simulink model "Passband_modulation_techniques"  (R2018b)
settings: Solver=VariableStepAuto  StartTime=0.0  StopTime=0.1  RelTol=1e-3  EnableMultiTasking=on
libraries: commfilt2 x6, commutil2 x5, commrandsrc3 x4, simulink x4
settings Model: Creator=hp  LastModifiedBy=HP
settings OptimizationCC: LifeSpan=inf
settings DebuggingCC: SFUnexpectedBacktrackingDiag=warning  SFNoUnconditionalDefaultTransitionDiag=warning
settings SFSimCC: SimUseLocalCustomCode=off
settings RTWCC: RTWUseLocalCustomCode=off
settings CodeAppCC: StateflowObjectComments=on
settings GRTTargetCC: TargetLangStandard=C89/C90 (ANSI)
settings ConfigComp: CovMetricSettings=dw  CovHtmlReporting=on  CovSaveCumulativeToWorkspaceVar=on  CovSaveSingleToWorkspaceVar=on  CovExternalEMLEnable=off

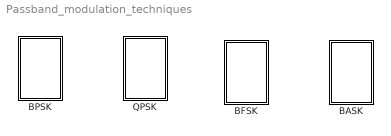
== system Passband_modulation_techniques ==
  BASK : Subsystem
  BFSK : Subsystem
  BPSK : Subsystem
  QPSK : Subsystem

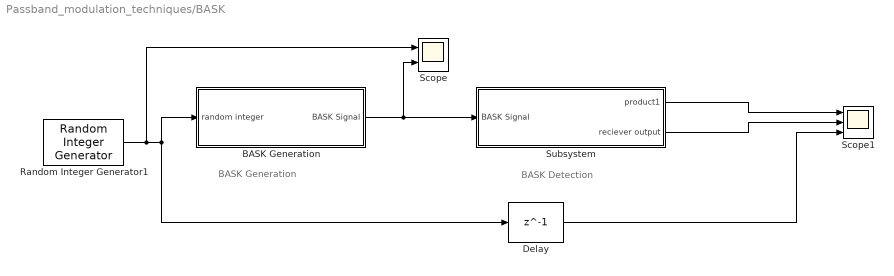
== system Passband_modulation_techniques/BASK ==
  note: BASK Detection
  note: BASK Generation
  BASK Generation : Subsystem
  Delay : Delay  DelayLength=1  InputProcessing=Columns as channels (frame based)
  Random Integer Generator1 : commrandsrc3/Random Integer Generator  SetSize=2  SeedSource=Auto  Seed=0  SampleTime=0.01  SamplesPerFrame=1  OutputDataType=double  SimulateUsing=Interpreted execution
  Scope : Scope  NumInputPorts=2
  Scope1 : Scope  NumInputPorts=3
  Subsystem : Subsystem
  wires:
  Subsystem/1(product1) -> Scope1/1
  Subsystem/2(reciever output) -> Scope1/2
  Delay/1 -> Scope1/3
  Random Integer Generator1/1 -> Scope/1, BASK Generation/1(random integer), Delay/1
  BASK Generation/1(BASK Signal) -> Scope/2, Subsystem/1(BASK Signal)

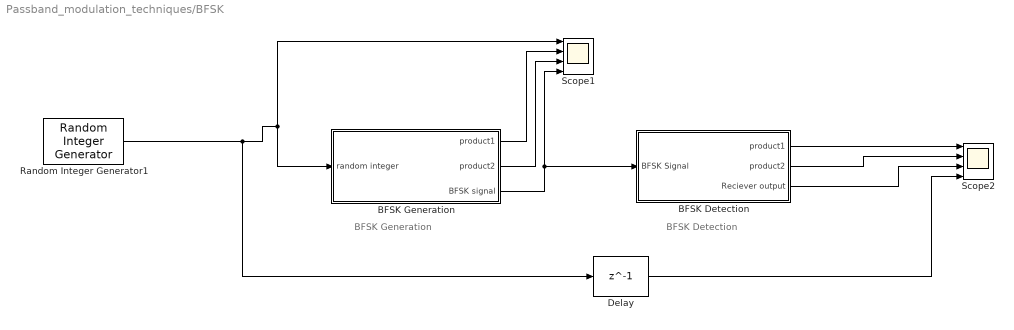
== system Passband_modulation_techniques/BFSK ==
  note: BFSK Detection
  note: BFSK Generation
  BFSK Detection : Subsystem
  BFSK Generation : Subsystem
  Delay : Delay  DelayLength=1  InputProcessing=Columns as channels (frame based)
  Random Integer Generator1 : commrandsrc3/Random Integer Generator  SetSize=2  SeedSource=Auto  Seed=0  SampleTime=0.01  SamplesPerFrame=1  OutputDataType=double  SimulateUsing=Interpreted execution
  Scope1 : Scope  NumInputPorts=4
  Scope2 : Scope  NumInputPorts=4
  wires:
  Random Integer Generator1/1 -> Delay/1, BFSK Generation/1(random integer), Scope1/1
  BFSK Generation/3(BFSK signal) -> Scope1/4, BFSK Detection/1(BFSK Signal)
  BFSK Generation/1(product1) -> Scope1/2
  BFSK Generation/2(product2) -> Scope1/3
  BFSK Detection/1(product1) -> Scope2/1
  BFSK Detection/2(product2) -> Scope2/2
  BFSK Detection/3(Reciever output) -> Scope2/3
  Delay/1 -> Scope2/4

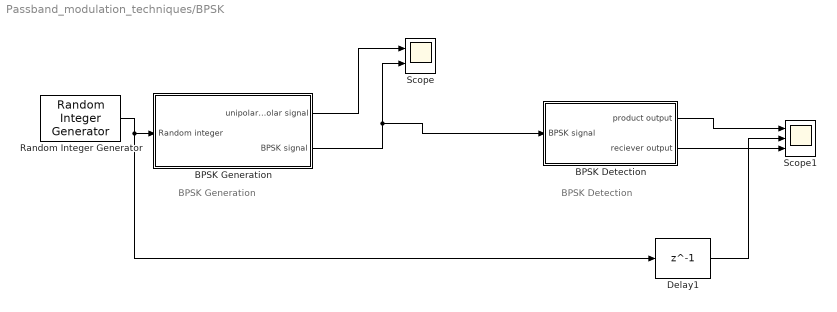
== system Passband_modulation_techniques/BPSK ==
  note: BPSK Generation
  note: BPSK Detection
  BPSK Detection : Subsystem
  BPSK Generation : Subsystem
  Delay1 : Delay  DelayLength=1  InputProcessing=Columns as channels (frame based)
  Random Integer Generator : commrandsrc3/Random Integer Generator  SetSize=2  SeedSource=Auto  Seed=0  SampleTime=0.01  SamplesPerFrame=1  OutputDataType=double  SimulateUsing=Interpreted execution
  Scope : Scope  NumInputPorts=2
  Scope1 : Scope  NumInputPorts=3
  wires:
  Random Integer Generator/1 -> Delay1/1, BPSK Generation/1(Random integer)
  BPSK Generation/2(BPSK signal) -> BPSK Detection/1(BPSK signal), Scope/2
  BPSK Generation/1(unipolar to bipolar signal) -> Scope/1
  BPSK Detection/1(product output) -> Scope1/1
  Delay1/1 -> Scope1/2
  BPSK Detection/2(reciever output) -> Scope1/3

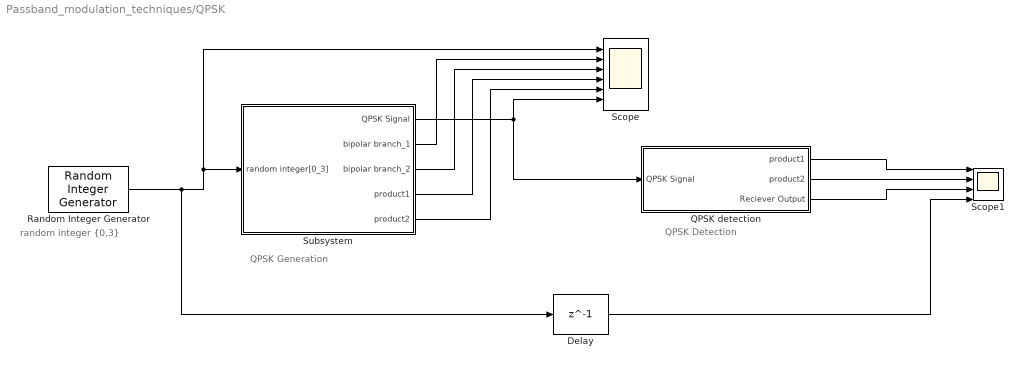
== system Passband_modulation_techniques/QPSK ==
  note: random integer {0,3}
  note: QPSK Generation
  note: QPSK Detection
  Delay : Delay  DelayLength=1  InputProcessing=Columns as channels (frame based)
  "QPSK detection " : Subsystem
  Random Integer Generator : commrandsrc3/Random Integer Generator  SetSize=4  SeedSource=Auto  Seed=0  SampleTime=0.01  SamplesPerFrame=1  OutputDataType=double  SimulateUsing=Interpreted execution
  Scope : Scope  NumInputPorts=6
  Scope1 : Scope  NumInputPorts=4
  Subsystem : Subsystem
  wires:
  Subsystem/1(QPSK Signal) -> Scope/6, "QPSK detection "/1(QPSK Signal)
  Random Integer Generator/1 -> Delay/1, Scope/1, Subsystem/1(random integer[0_3])
  "QPSK detection "/1(product1) -> Scope1/1
  "QPSK detection "/2(product2) -> Scope1/2
  "QPSK detection "/3(Reciever Output) -> Scope1/3
  Delay/1 -> Scope1/4
  Subsystem/2(bipolar branch_1) -> Scope/2
  Subsystem/3(bipolar branch_2) -> Scope/3
  Subsystem/4(product1) -> Scope/4
  Subsystem/5(product2) -> Scope/5

== system Passband_modulation_techniques/BASK/BASK Generation ==
  random integer : Inport
  Product2 : Product
  Sine Wave1 : Sin  Frequency=300*2*pi  Phase=pi/2  SampleTime=1/(300*100)
  BASK Signal : Outport
  wires:
  random integer/1 -> Product2/1
  Sine Wave1/1 -> Product2/2
  Product2/1 -> BASK Signal/1

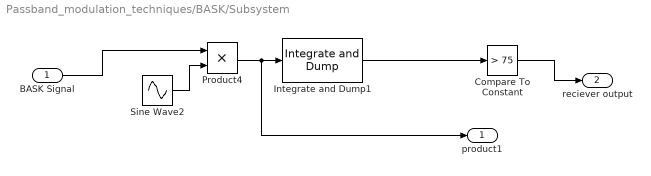
== system Passband_modulation_techniques/BASK/Subsystem ==
  BASK Signal : Inport
  Compare To Constant : simulink/Logic and Bit Operations/Compare To Constant  relop=>  const=75  OutDataTypeStr=boolean
  Integrate and Dump1 : commfilt2/Integrate and Dump  obssamples=300  offsetsamples=0  nodump=off  roundingMode=Floor  overflowMode=off  outputDataTypeStr=Inherit: Same as accumulator  outputLastDataTypeStr=Inherit: Same as accumulator
  Product4 : Product
  Sine Wave2 : Sin  Frequency=300*2*pi  Phase=pi/2  SampleTime=1/(300*100)
  product1 : Outport
  reciever output : Outport  Port=2
  wires:
  Sine Wave2/1 -> Product4/2
  BASK Signal/1 -> Product4/1
  Product4/1 -> product1/1, Integrate and Dump1/1
  Integrate and Dump1/1 -> Compare To Constant/1
  Compare To Constant/1 -> reciever output/1

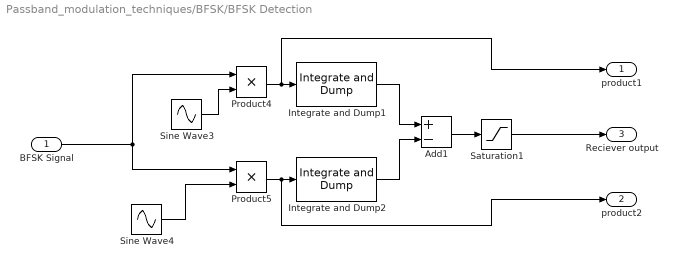
== system Passband_modulation_techniques/BFSK/BFSK Detection ==
  BFSK Signal : Inport
  Add1 : Sum  Inputs=+-
  Integrate and Dump1 : commfilt2/Integrate and Dump  obssamples=300  offsetsamples=0  nodump=off  roundingMode=Floor  overflowMode=off  outputDataTypeStr=Inherit: Same as accumulator  outputLastDataTypeStr=Inherit: Same as accumulator
  Integrate and Dump2 : commfilt2/Integrate and Dump  obssamples=300  offsetsamples=0  nodump=off  roundingMode=Floor  overflowMode=off  outputDataTypeStr=Inherit: Same as accumulator  outputLastDataTypeStr=Inherit: Same as accumulator
  Product4 : Product
  Product5 : Product
  Saturation1 : Saturate  UpperLimit=1  LowerLimit=0
  Sine Wave3 : Sin  Frequency=300*2*pi  Phase=pi/2  SampleTime=1/(600*50)
  Sine Wave4 : Sin  Frequency=600*2*pi  Phase=pi/2  SampleTime=1/(600*50)
  product1 : Outport
  product2 : Outport  Port=2
  Reciever output : Outport  Port=3
  wires:
  Saturation1/1 -> Reciever output/1
  Integrate and Dump1/1 -> Add1/1
  BFSK Signal/1 -> Product4/1, Product5/1
  Sine Wave4/1 -> Product5/2
  Sine Wave3/1 -> Product4/2
  Product5/1 -> product2/1, Integrate and Dump2/1
  Integrate and Dump2/1 -> Add1/2
  Product4/1 -> product1/1, Integrate and Dump1/1
  Add1/1 -> Saturation1/1

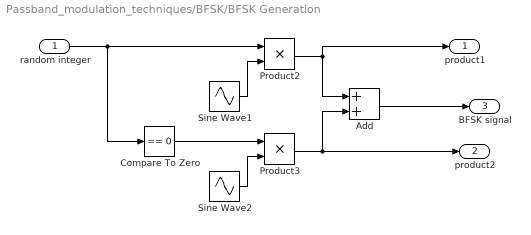
== system Passband_modulation_techniques/BFSK/BFSK Generation ==
  random integer : Inport
  Add : Sum
  Compare To Zero : simulink/Logic and Bit Operations/Compare To Zero  relop===  OutDataTypeStr=boolean
  Product2 : Product
  Product3 : Product
  Sine Wave1 : Sin  Frequency=300*2*pi  Phase=pi/2  SampleTime=1/(600*50)
  Sine Wave2 : Sin  Frequency=600*2*pi  Phase=pi/2  SampleTime=1/(600*50)
  product1 : Outport
  product2 : Outport  Port=2
  BFSK signal : Outport  Port=3
  wires:
  Sine Wave2/1 -> Product3/2
  Product2/1 -> Add/1, product1/1
  Add/1 -> BFSK signal/1
  Sine Wave1/1 -> Product2/2
  random integer/1 -> Compare To Zero/1, Product2/1
  Product3/1 -> Add/2, product2/1
  Compare To Zero/1 -> Product3/1

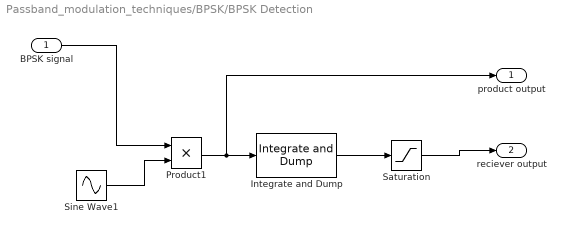
== system Passband_modulation_techniques/BPSK/BPSK Detection ==
  BPSK signal : Inport
  Integrate and Dump : commfilt2/Integrate and Dump  obssamples=150  offsetsamples=0  nodump=off  roundingMode=Floor  overflowMode=off  outputDataTypeStr=Inherit: Same as accumulator  outputLastDataTypeStr=Inherit: Same as accumulator
  Product1 : Product
  Saturation : Saturate  UpperLimit=1  LowerLimit=0
  Sine Wave1 : Sin  Frequency=300*2*pi  SampleTime=1/(300*50)
  product output : Outport
  reciever output : Outport  Port=2
  wires:
  Sine Wave1/1 -> Product1/2
  Product1/1 -> product output/1, Integrate and Dump/1
  BPSK signal/1 -> Product1/1
  Integrate and Dump/1 -> Saturation/1
  Saturation/1 -> reciever output/1

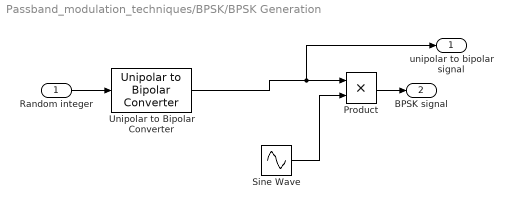
== system Passband_modulation_techniques/BPSK/BPSK Generation ==
  Random integer : Inport
  Product : Product
  Sine Wave : Sin  Frequency=300*2*pi  SampleTime=1/(300*50)
  Unipolar to Bipolar Converter : commutil2/Unipolar to Bipolar Converter  M=2  polarity=Positive  dataType=Inherit via internal rule
  unipolar to bipolar signal : Outport
  BPSK signal : Outport  Port=2
  wires:
  Unipolar to Bipolar Converter/1 -> unipolar to bipolar signal/1, Product/1
  Sine Wave/1 -> Product/2
  Random integer/1 -> Unipolar to Bipolar Converter/1
  Product/1 -> BPSK signal/1

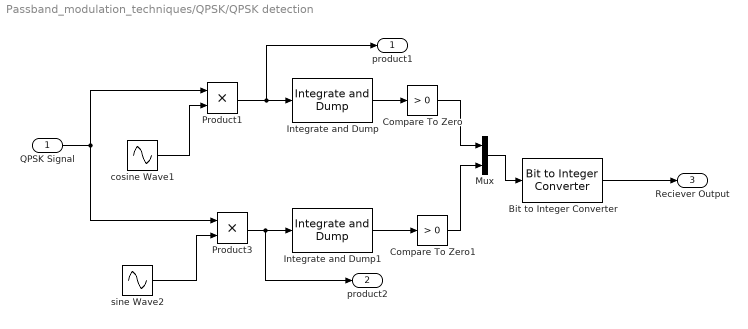
== system Passband_modulation_techniques/QPSK/QPSK detection  ==
  QPSK Signal : Inport
  Bit to Integer Converter : commutil2/Bit to Integer Converter  nbits=2  bitOrder=MSB first  signedOutputValues=Unsigned  outDtype=Inherit via internal rule  outDtypeSigned=Inherit via internal rule
  Compare To Zero : simulink/Logic and Bit Operations/Compare To Zero  relop=>  OutDataTypeStr=boolean
  Compare To Zero1 : simulink/Logic and Bit Operations/Compare To Zero  relop=>  OutDataTypeStr=boolean
  Integrate and Dump : commfilt2/Integrate and Dump  obssamples=300  offsetsamples=0  nodump=off  roundingMode=Floor  overflowMode=off  outputDataTypeStr=Inherit: Same as accumulator  outputLastDataTypeStr=Inherit: Same as accumulator
  Integrate and Dump1 : commfilt2/Integrate and Dump  obssamples=300  offsetsamples=0  nodump=off  roundingMode=Floor  overflowMode=off  outputDataTypeStr=Inherit: Same as accumulator  outputLastDataTypeStr=Inherit: Same as accumulator
  Mux : Mux  Inputs=2
  Product1 : Product
  Product3 : Product
  cosine Wave1 : Sin  Amplitude=0.7071  Frequency=300*2*pi  Phase=pi/2  SampleTime=1/(300*100)
  sine Wave2 : Sin  Amplitude=0.7071  Frequency=300*2*pi  SampleTime=1/(300*100)
  product1 : Outport
  product2 : Outport  Port=2
  Reciever Output : Outport  Port=3
  wires:
  Product3/1 -> product2/1, Integrate and Dump1/1
  Mux/1 -> Bit to Integer Converter/1
  Product1/1 -> product1/1, Integrate and Dump/1
  QPSK Signal/1 -> Product1/1, Product3/1
  Integrate and Dump/1 -> Compare To Zero/1
  Compare To Zero1/1 -> Mux/2
  cosine Wave1/1 -> Product1/2
  Integrate and Dump1/1 -> Compare To Zero1/1
  sine Wave2/1 -> Product3/2
  Compare To Zero/1 -> Mux/1
  Bit to Integer Converter/1 -> Reciever Output/1

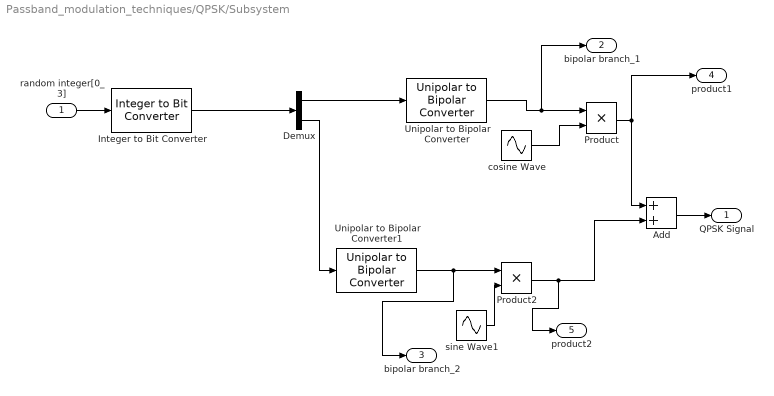
== system Passband_modulation_techniques/QPSK/Subsystem ==
  random integer[0_3] : Inport
  Add : Sum
  Demux : Demux  Outputs=2
  Integer to Bit Converter : commutil2/Integer to Bit Converter  nbits=2  signedInputValues=Unsigned  bitOrder=MSB first  outDtype=Inherit via internal rule
  Product : Product
  Product2 : Product
  Unipolar to Bipolar Converter : commutil2/Unipolar to Bipolar Converter  M=2  polarity=Positive  dataType=Inherit via internal rule
  Unipolar to Bipolar Converter1 : commutil2/Unipolar to Bipolar Converter  M=2  polarity=Positive  dataType=Inherit via internal rule
  cosine Wave : Sin  Amplitude=0.7071  Frequency=300*2*pi  Phase=pi/2  SampleTime=1/(300*100)
  sine Wave1 : Sin  Amplitude=0.7071  Frequency=300*2*pi  SampleTime=1/(300*100)
  QPSK Signal : Outport
  bipolar branch_1 : Outport  Port=2
  bipolar branch_2 : Outport  Port=3
  product1 : Outport  Port=4
  product2 : Outport  Port=5
  wires:
  Unipolar to Bipolar Converter/1 -> bipolar branch_1/1, Product/1
  Product2/1 -> product2/1, Add/2
  sine Wave1/1 -> Product2/2
  cosine Wave/1 -> Product/2
  Product/1 -> product1/1, Add/1
  Demux/1 -> Unipolar to Bipolar Converter/1
  Demux/2 -> Unipolar to Bipolar Converter1/1
  Unipolar to Bipolar Converter1/1 -> bipolar branch_2/1, Product2/1
  Integer to Bit Converter/1 -> Demux/1
  Add/1 -> QPSK Signal/1
  random integer[0_3]/1 -> Integer to Bit Converter/1
